simulink model "Solver"  (R2016b)
settings: Solver=ode4  StartTime=0.0  StopTime=Inf  FixedStep=base_dT  RelTol=1e-3
values from neighbouring files (symbols this model uses):
  base_dT = Simulink.Parameter    [SolverInit.m]
  E2C_bEgoFol = Simulink.Parameter    [SolverInit.m]
  E2C_bUseCollo = Simulink.Parameter    [SolverInit.m]
  E2C_c2_dTB = Simulink.Parameter    [SolverInit.m]
  E2C_c_dTB = Simulink.Parameter    [SolverInit.m]
  E2C_d_HDW1 = Simulink.Parameter    [SolverInit.m]
  E2C_d_HDW2 = Simulink.Parameter    [SolverInit.m]
  E2C_DeltaT = Simulink.Parameter    [SolverInit.m]
  E2C_df_term = Simulink.Parameter    [SolverInit.m]
  E2C_dz_term = Simulink.Parameter    [SolverInit.m]
  E2C_Max_iter = Simulink.Parameter    [SolverInit.m]
  E2C_t_HDW1 = Simulink.Parameter    [SolverInit.m]
  E2C_t_HDW2 = Simulink.Parameter    [SolverInit.m]
  E2C_T_TB_thr = Simulink.Parameter    [SolverInit.m]
  E2C_tiSolverPeriod_C = Simulink.Parameter    [SolverInit.m]
  E2C_U_max = Simulink.Parameter    [SolverInit.m]
  E2C_U_min = Simulink.Parameter    [SolverInit.m]
  E2C_V_max = Simulink.Parameter    [SolverInit.m]
  E2C_V_min = Simulink.Parameter    [SolverInit.m]
  E2C_w_delta_u = Simulink.Parameter    [SolverInit.m]
  E2C_w_epsilon_lin = Simulink.Parameter    [SolverInit.m]
  E2C_weight_TTB = Simulink.Parameter    [SolverInit.m]
  Inp_mf_exh_par = Simulink.Parameter    [SolverInit.m]
  Inp_t_eu_par = Simulink.Parameter    [SolverInit.m]
  NP_trial = Simulink.Parameter    [SolverInit.m]
  t_EndSimulation = Simulink.Parameter    [SolverInit.m]
  t_StartSimulation = Simulink.Parameter    [SolverInit.m]
libraries: simulink x3, dspsigops x2
(part 2 of 2)

== matlab function Solver/QP Runner/MATLAB Function - MPC ==
  data: NP input; v_ input; p_ input; T_TB_ input; U_OUTPUT output; v_lead_s input; p_lead input; v_lead input; V_OUTPUT output double; z_laststep input size=[41 1]; z_new output size=[41 1]; w_epsilon input; weight_TTB input; iA0 input boolean size=[NP_trial*6+2,1] [1..250]; t_StartSimulation input; V_lim input; U_lim input; d_HDW input; t_HDW input; w_epsilon_lin input; T_TB_thr input; EgoFol input; UseCollo input; c_dTB input; c2_dTB input; w_delta_u input; t_ input; iA1 output; Inp_mf_exh_par parameter; Inp_t_eu_par parameter; v_0 output size=[40 1]; TTB_0 output size=[40 1]; f_nonl_new output; delta_f output size=[1 1]
function [U_OUTPUT,V_OUTPUT,z_new,iA1,v_0,TTB_0,f_nonl_new,delta_f]    = ...
    NLMPC_TB_Intern_Fcn(NP,v_,p_,T_TB_,v_lead_s,p_lead,v_lead,z_laststep,...
    w_epsilon,weight_TTB,iA0,t_StartSimulation,V_lim,U_lim,d_HDW,t_HDW,w_epsilon_lin,T_TB_thr,EgoFol,UseCollo,...
    c_dTB,c2_dTB,w_delta_u,t_,...
    Inp_mf_exh_par,Inp_t_eu_par)
% 06/29
% change tau_{TB} to c_dTB/(meu+c2_dTB)

%%
% ------------ Load maps  ---------------------------------
Inp.Vspeed = [0:0.1:30]; 
% delta_v = 0.4 does not work!
Inp.Acce = [-6:0.1:6]'; % repmat([-6:0.1:6]',1,351);
Inp.mf_exh = Inp_mf_exh_par; % (1:4:end,1:2:end);
Inp.t_eu = Inp_t_eu_par; % (1:4:end,1:2:end);
% coder.extrinsic('quadprog'); 
% % Option 2:
% % do not use collocation!
% 
if true

%t_ = 0.0;  % not used in testing case. 

assert (NP <= 50);
% assert (NP_trial <= 50);

% persistent PARS
PARS.NP = 40;
PARS.dT = 1;
PARS.weight_a = 1;
PARS.ConstraintCase = 'soft'; % or 'hard' is the same
PARS.t_StartSimulation = t_StartSimulation;

% % ------------ parameters ----------------------------------------------
PARS.V_lim = V_lim;   % inputs from matlab
PARS.U_lim = U_lim;   % inputs from matlab
PARS.d_HDW = d_HDW;   % inputs from matlab
PARS.t_HDW = t_HDW;   % inputs from matlab
PARS.w_epsilon_lin = w_epsilon_lin;
PARS.w_epsilon = w_epsilon;
PARS.T_TB_thr = T_TB_thr;   % 240
PARS.c_dTB = c_dTB;   %3.3
PARS.c2_dTB = c2_dTB;
PARS.w_delta_u = w_delta_u;   % cost on delta_u, originally 0



n = 3; % length(x_)
m = 1; % size(u_past);
Ndec = n + m*(PARS.NP) +1; % [x_,u_opt,t_]
Nz = 3*PARS.NP+1; % z=[du(0),...du(NP-1),dv(1),...,dv(NP),dT(1),...,dT(NP),d_epsilon]



% % ------------ Preview ------------------------------------------------


v_ref = [v_lead_s(1:PARS.NP);v_lead_s(PARS.NP)];
if abs(v_lead-v_ref(1))>1e-6
v_ref(1) = v_lead;
end

z_new = zeros(41,1);

    
acce_ref = (v_ref(2:end)-v_ref(1:end-1))/PARS.dT;
dist_ref = zeros(PARS.NP+1,1);
% coder.varsize('dist_ref', [50,1]); % this is the preview

% initialize

x_ = [v_,p_,T_TB_]';
%coder.extrinsic('linprog'); 
% coder.extrinsic('qinterp2');
% coder.extrinsic('qinterp2_eval');
% coder.extrinsic('tic')
% coder.extrinsic('toc')

% ------------ If do not start optimization -------------------------
if EgoFol==0 || t_<=t_StartSimulation
    U_OUTPUT = 0;
    U_OUTPUT = min(PARS.U_lim(2),(v_lead-v_)/PARS.dT); % track the lead speed% acce_ref(1);
    V_OUTPUT = 0;
    V_OUTPUT = v_ref(1);
    iA1 = false(242,1);     % false(40*4+40*2+2,1);
    z_new = [ones(40,1);0];
    v_0 = v_ref(1:40);
    TTB_0 = 150+0*v_0;
    f_nonl_new = 100;
    delta_f = 0;
else
    % ------------ CREATE DISTANCE BOUNDS ---------------------------------

    dist_ref(1) = p_lead;
    A3t = zeros(PARS.NP);
    for i=1:PARS.NP
        A3t(i:PARS.NP,i) = [1:PARS.NP-i+1]-0.5;
    end
    Aineq3 = [ [PARS.dT:PARS.dT:PARS.NP*PARS.dT]', ones(PARS.NP,1), zeros(PARS.NP,n-2), A3t*PARS.dT^2 ,zeros(PARS.NP,1)];
    dist_ref(2:PARS.NP+1) = Aineq3*[[v_ref(1);p_lead;0];acce_ref;0];
    dist_hi_ref = dist_ref - PARS.d_HDW(1);
    dist_lo_ref = dist_ref - PARS.d_HDW(2);

    % --------------- Optimization reference ------------------------------
    z_cur_2 = z_laststep;    % z_cur_2 should be the guessed z_curr step, from either z_curr-1 or from last sqp iteration.
    
    z_cur = zeros(45,1);      % zeros(3+40+1+1,1);
    z_cur = [x_;z_cur_2(1:PARS.NP);t_;z_cur_2(PARS.NP+1)];
    
    % ----------- reference Acceleration -----------------------------------------
    % if max(TTB_laststep)<=150.1 && min(TTB_laststep)>=149.9
    u_opt = zeros(40,1);
    u_opt = z_cur_2(1:PARS.NP);
    u_opt(u_opt>PARS.U_lim(2)) = PARS.U_lim(2);
    u_opt(u_opt<PARS.U_lim(1)) = PARS.U_lim(1);
    z_cur_2(1:PARS.NP) = u_opt;
    v_opt = zeros(40,1);
    % v_opt = v(curr+1:curr+NP)
    Aineq1 = [ones(PARS.NP,1),zeros(PARS.NP,n-1),PARS.dT*tril(ones(PARS.NP,PARS.NP),0),zeros(PARS.NP,1)];
    v_opt = Aineq1*z_cur(1:n+PARS.NP+1);
    v_opt(v_opt<PARS.V_lim(1))=PARS.V_lim(1);
    v_opt(v_opt>PARS.V_lim(2))=PARS.V_lim(2);

    u_opt = (v_opt-[v_;v_opt(1:40-1)])/PARS.dT;
    u_opt(u_opt>PARS.U_lim(2)) = PARS.U_lim(2);
    u_opt(u_opt<PARS.U_lim(1)) = PARS.U_lim(1);
    v_0 = zeros(40,1); 
    v_0(1:PARS.NP) = [max(min(v_,PARS.V_lim(2)),PARS.V_lim(1));v_opt(1:PARS.NP-1)];  % nominal v at t(curr:curr+NP-1)
    
    % ------------ Hession ------------ 
    % add cost on sum(delta_u) 06/17/2019
    H_delta_u = zeros(PARS.NP+1);
    H_delta_u(1,1) = 1 *2*PARS.w_delta_u;
    H_delta_u(PARS.NP,PARS.NP) = 1 *2*PARS.w_delta_u;
    for i = 2:PARS.NP-1
        H_delta_u(i,i) = 2 * 2*PARS.w_delta_u;
        H_delta_u(i-1,i) = -1 * 2*PARS.w_delta_u;
        H_delta_u(i,i-1) = -1 * 2*PARS.w_delta_u;
    end
    H_delta_u(PARS.NP-1,PARS.NP) = -1 * 2*PARS.w_delta_u;
    H_delta_u(PARS.NP,PARS.NP-1) = -1 * 2*PARS.w_delta_u;
    
    % ------------ calculate the cost before opt ------------ 
    ind1 = 0.0*zeros(40,1); %(0*v_0)*zeros(1,4);
    ind2 = 0.0*zeros(40,1);
    ind3 = 0.0*zeros(40,1);
    ind4 = 0.0*zeros(40,1);
    dfxi = 0.0*zeros(40,1); % (0*v_0)*zeros(1,2);
    dfyi = 0.0*zeros(40,1); % (0*v_0)*zeros(1,2);
    flagIn = zeros(40,1); % 0*v_0;
    % [ind,dfxy,flagIn] = qinterp2(Inp.Vspeed, Inp.Acce, v_0, u_opt, 2);
    %% This section is qinterp2.m
%     X = Inp.Vspeed;
%     Y = Inp.Acce;
    xi = v_0;
    yi = u_opt;
    librarySize = [0 0];
    librarySize = [length(Inp.Acce),length(Inp.Vspeed)];
    ndx = 0.0;  ndy = 0.0;
    ndx = 1/(Inp.Vspeed(1,2)-Inp.Vspeed(1,1));    
    ndy = 1/(Inp.Acce(2,1)-Inp.Acce(1,1));
    % Begin mapping xi and yi vectors onto index space by subtracting library
    % array minima and scaling to index spacing
    xi(xi>=Inp.Vspeed(1,end)) = Inp.Vspeed(1,end)-1e-8*(Inp.Vspeed(1,end)-Inp.Vspeed(1,1));
    yi(yi>=Inp.Acce(end,1)) = Inp.Acce(end,1)-1e-8*(Inp.Acce(end,1)-Inp.Acce(1,1));

    xi = (xi - Inp.Vspeed(1,1))*ndx;       yi = (yi - Inp.Acce(1,1))*ndy;
    fxi = floor(xi)+1;  fyi = floor(yi)+1;   % x_i and y_i
    dfxi = xi-fxi+1;    dfyi = yi-fyi+1;     % Location in unit square

    % flagIn determines whether the requested location is inside of the
    % library arrays
    flagIn = fxi>0 & fxi<librarySize(2) & ~isnan(fxi) &...
        fyi>0 & fyi<librarySize(1) & ~isnan(fyi);
%     if min(flagIn)==0
%         1+1
%         flagIn
%     end
    % Toss all out-of-bounds variables now to save time
    fxi = fxi(flagIn); fyi = fyi(flagIn);
    dfxi = dfxi(flagIn); dfyi = dfyi(flagIn);

    % Find bounding vertices
    ind1 = fyi + librarySize(1)*(fxi-1);     % Indices of (  x_i  ,  y_i  )
    ind2 = fyi + librarySize(1)*fxi;         % Indices of ( x_i+1 ,  y_i  )
    ind3 = fyi + 1 + librarySize(1)*fxi;     % Indices of ( x_i+1 , y_i+1 )
    ind4 = fyi + 1 + librarySize(1)*(fxi-1); % Indices of (  x_i  , y_i+1 )


    flagIn = double(flagIn);

    %%

    TTB_0 = zeros(40,1);
    TTB_0(1:PARS.NP) = [x_(3); zeros(PARS.NP-1,1)];
    meu_0 = zeros(40,1);
    Tin_0 = zeros(40,1);

    % meu_0 = qinterp2_eval(Inp.mf_exh, ind,dfxy,flagIn);
    % Tin_0 = qinterp2_eval(Inp.t_eu, ind,dfxy,flagIn);
    %% This is for qinterp2_eval.m
    Z = Inp.mf_exh; 
    Zi = 0.0*ind1;
    Zi(find(flagIn==1)) = Z(ind1).*(1-dfxi).*(1-dfyi) + ...
        Z(ind2).*dfxi.*(1-dfyi) + ...
        Z(ind4).*(1-dfxi).*dfyi + ...
        Z(ind3).*dfxi.*dfyi;
    meu_0 = Zi;
    % derivatives
%     p_meu_p_u = qinterp2_eval(Inp.mf_exh_pu, ind,dfxy,flagIn);
%     p_meu_p_x = qinterp2_eval(Inp.mf_exh_px, ind,dfxy,flagIn);
    p_meu_p_u = 0.0*v_0;
    p_meu_p_x = 0.0*v_0;
    p_meu_p_u = (Z(ind4)-Z(ind1)).*(1-dfxi)*ndy + ...
        (Z(ind3)-Z(ind2)).*(dfxi)*ndy;
    p_meu_p_x = (Z(ind2)-Z(ind1))*ndx.*(1-dfyi) + ...
        (Z(ind3)-Z(ind4))*ndx.*(dfyi);

    Z = Inp.t_eu; 
    Zi(find(flagIn==1)) = Z(ind1).*(1-dfxi).*(1-dfyi) + ...
        Z(ind2).*dfxi.*(1-dfyi) + ...
        Z(ind4).*(1-dfxi).*dfyi + ...
        Z(ind3).*dfxi.*dfyi;
    Tin_0 = Zi;
    % derivatives
%     p_Teu_p_u = qinterp2_eval(Inp.t_eu_pu, ind,dfxy,flagIn);
%     p_Teu_p_x = qinterp2_eval(Inp.t_eu_px, ind,dfxy,flagIn);
    p_Teu_p_u = 0.0*v_0;
    p_Teu_p_x = 0.0*v_0;
    p_Teu_p_u = (Z(ind4)-Z(ind1)).*(1-dfxi)*ndy + ...
        (Z(ind3)-Z(ind2)).*(dfxi)*ndy;
    p_Teu_p_x = (Z(ind2)-Z(ind1))*ndx.*(1-dfyi) + ...
        (Z(ind3)-Z(ind4))*ndx.*(dfyi);

    %%
%     for i = 1:PARS.NP-1
%         TTB_0(i+1,1) = TTB_0(i,1) + PARS.dT.*meu_0(i,1)/PARS.c_dTB.*(Tin_0(i,1)-TTB_0(i,1));
%     end
    for i = 1:PARS.NP-1
        TTB_0(i+1,1) = TTB_0(i,1) + PARS.dT.*(meu_0(i,1)+PARS.c2_dTB)/PARS.c_dTB.*(Tin_0(i,1)-TTB_0(i,1));
    end
    
    f_nonl = 0; % compute the actual cost value
    f_nonl = u_opt'*eye(PARS.NP)*u_opt + ...
        (1e-3*weight_TTB)*sum(double(TTB_0<PARS.T_TB_thr).*(TTB_0-PARS.T_TB_thr).^2) + ...
        PARS.w_epsilon*(z_cur_2(PARS.NP+1))^2 + ...
        PARS.w_epsilon_lin*(z_cur_2(PARS.NP+1)) + ...
        0.5*u_opt'*H_delta_u(1:PARS.NP,1:PARS.NP)*u_opt;
    
    % ------------ Create NLMPC Aeq,Beq ------------------------------------
    Aeq = zeros(n, Ndec);
    beq = zeros(n, 1);
    Aeq(1:n, 1:n) = eye(n);
    beq(1:n) = x_;

    % ------------ Create NLMPC Aineq,Bineq ------------------------------------
    Aineq1 = [ones(PARS.NP,1),zeros(PARS.NP,n-1),PARS.dT*tril(ones(PARS.NP,PARS.NP),0),zeros(PARS.NP,1)];
    bineq1 = V_lim(2)-0.001+zeros(PARS.NP,1);
    Aineq2 = -Aineq1;
    bineq2 = -(V_lim(1)-0.001)+zeros(PARS.NP,1);
    % Aineq3 already defined above
    bineq3 = dist_hi_ref(2:PARS.NP+1);
    Aineq4 = -Aineq3;
    bineq4 = -( dist_lo_ref(2:PARS.NP+1) );
    Aineq5 = [];
    bineq5 = [];

    
%     AINEQ = [[Aineq1;Aineq2;Aineq3+PARS.t_HDW(1)*Aineq1;Aineq4-PARS.t_HDW(2)*Aineq1;Aineq5],...
%         [-1e-5*ones(2*length(Aineq1(:,1)),1);-ones(2*length(Aineq1(:,1)),1);zeros(length(bineq5),1)]];
%     BINEQ = [bineq1;bineq2;bineq3;bineq4;bineq5];

    % ----------- Create NLMPC lb,ub -----------------------------------------
    lb = zeros(3 + 40 +1,1);
    ub = zeros(3 + 40 +1,1);
    lb(end) = t_;
    ub(end) = t_;
    lb(1:3) = x_;
    ub(1:3) = x_;
    lb(1+3:3+40) = PARS.U_lim(1);
    ub(1+3:3+40) = PARS.U_lim(2);

    % ----------- Create Initial guess -----------------------------------------
%     if iter ==0
%         z_last = zeros(40+1,1);  %initial guess.  n+PARS.NP+1
%         for i = 1:40
%             z_last(i) = interp1([-0.1;t_laststep;20000],[0;u_laststep;0],t_+i-1);
%         end
%         z_last(40+1) = 0;  
%         z_laststep = z_last; 
%     else
%         % z_laststep = z_laststep; % in the same sqp, not same qp.
%     end
    % --------------- Optimization reference ------------------------------
    Hession_f1 = 2* 1*diag([ones(1,PARS.NP), PARS.w_epsilon ]) + H_delta_u; % a^2+epsilon^2part
    
    

    % ----------- calculate gradient ------------------
    % grad_z(f)
    % we need 

    

%     % ---------------------finite differentence calculating gradiant ---------------
%     du = 0.001;
%     delta_u = du*ones(40,1);  % perturbation of u
%     V_pert = zeros(40,40);
%     % V_pert = v_{0:NP-1}(u^0+du(0)),v_{0:NP-1}(u^0+du(1)),...,v_{0:NP-1}(u^0+du(NP-1))
%     % first column, perturb du(0),affect 2:NP;
%     % second column, perturb du(1),affect 3:NP;
%     % last column, perturb du(1)
%     V_pert = [[1,zeros(1,n+PARS.NP-1)];Aineq1(1:PARS.NP-1,1:n+PARS.NP)]*[x_*(1+0*u_opt');u_opt*(1+0*u_opt')+diag(delta_u)];
%     V_pert=max(V_pert,0);
%     V_pert=min(V_pert,30);
%     V_ppert = V_pert*2- v_0*(1+0*v_0');
%     V_ppert = v_{0:NP-1}(u^0+2du(0)),v_{0:NP-1}(u^0+2du(1)),...,v_{0:NP-1}(u^0+2du(NP-1))
%         TTB_pert = zeros(40,40);
%         TTB_pert = TTB_0*(1+0*TTB_0');  % upper right small triangle is equal to TTB_0.
% 
%         for i = 1:PARS.NP-1
%             u_pert = u_opt*0;
%             u_pert = u_opt;
%             u_pert(i) = u_pert(i)+du;
%             ind_i = zeros(40-i+1,4); %(0*v_0)*zeros(1,4);
%             dfxy_i = zeros(40-i+1,2); % (0*v_0)*zeros(1,2);
%             flagIn_i = zeros(40-i+1,1); % 0*v_0;
% 
%             [ind_i,dfxy_i,flagIn_i] = qinterp2(Inp.Vspeed, Inp.Acce, V_pert(i:PARS.NP,i), u_pert(i:PARS.NP), 2);
%             meu_i = zeros(40-i+1,1);
%             meu_i = qinterp2_eval(Inp.mf_exh, ind_i,dfxy_i,flagIn_i );
%             Tin_i = zeros(40-i+1,1);
%             Tin_i = qinterp2_eval(Inp.t_eu, ind_i,dfxy_i,flagIn_i );
%             for j = i:PARS.NP-1
%                 TTB_pert(j+1,i) = TTB_pert(j,i)+PARS.dT.*meu_i(j-(i-1))/3.3.*(Tin_i(j-(i-1))-TTB_pert(j,i));
%             end
%         end
%         grad_f2_p1 = [0*delta_u;0]*(0*delta_u)';
%         grad_f2_p1(1:PARS.NP,1:PARS.NP) = ((TTB_pert-TTB_0*(1+0*TTB_0'))/du)';
%         grad_f2_p2 = 0*delta_u;
%         grad_f2_p2 = (1e-3*weight_TTB)*(TTB_0-240).*(TTB_0<240);
%         grad_f2 = [0*delta_u;0];
%         grad_f2 = grad_f2_p1*grad_f2_p2;
%         Hession_f2 = [0*delta_u;0]*[0*delta_u;0]';
%         Hession = Hession_f1+Hession_f2;
%         grad_f1 = Hession_f1*z_cur_2;
%         grad_f = 0*grad_f1;
%         grad_f = grad_f1 + grad_f2;
%     
    % --------------------- direct calculating gradiant ---------------
    
    Hession_f2 = [0*v_0;0]*[0*v_0;0]';
    Hession = Hession_f1 + Hession_f2; %0.5*z'*H*z!!
    grad_f1 = Hession_f1*z_cur_2 + [0*v_0;PARS.w_epsilon_lin];
    


    %%
%     d_TTB_plus_d_z = PARS.dT/PARS.c_dTB*( p_Teu_p_u.*meu_0 + (Tin_0-TTB_0).*p_meu_p_u ); % PARS.c_dTB = 3.3
%     d_TTB_plus_d_z(PARS.NP) = 0;
%     p_TTB_plus_p_x = PARS.dT/PARS.c_dTB*( p_Teu_p_x.*meu_0 + (Tin_0-TTB_0).*p_meu_p_x );
%     p_TTB_plus_p_x(PARS.NP) = 0;
%     p_TTB_plus_p_TTB = 1-PARS.dT/PARS.c_dTB*meu_0;
%     p_TTB_plus_p_TTB(PARS.NP) = 0;
    
    d_TTB_plus_d_z = PARS.dT*( p_Teu_p_u.*(meu_0+PARS.c2_dTB)/PARS.c_dTB + (Tin_0-TTB_0).*p_meu_p_u/PARS.c_dTB ); % PARS.c_dTB = 3.3
    d_TTB_plus_d_z(PARS.NP) = 0;
    p_TTB_plus_p_x = PARS.dT*( p_Teu_p_x.*(meu_0+PARS.c2_dTB)/PARS.c_dTB + (Tin_0-TTB_0).*p_meu_p_x/PARS.c_dTB );
    p_TTB_plus_p_x(PARS.NP) = 0;
    p_TTB_plus_p_TTB = 1-PARS.dT/PARS.c_dTB*(meu_0+PARS.c2_dTB);
    p_TTB_plus_p_TTB(PARS.NP) = 0;
    
    
    d_TTB_d_z = 0*v_0*[0*v_0;0]'; % NP*(NP+1)
    for i = 1:PARS.NP-1 % i is the row
        d_TTB_d_z(i+1,i) = d_TTB_plus_d_z(i);
    end
    
    for i = 3:PARS.NP % i is the row
        d_TTB_d_z(i,1:i-2) = PARS.dT*p_TTB_plus_p_x(i-1) + d_TTB_d_z(i-1,1:i-2)*p_TTB_plus_p_TTB(i-1);
    end
    
    grad_f2_p2 = 2*(1e-3*weight_TTB)*(TTB_0-240).*(double(TTB_0<240));  % changed to ("2*") 06062019
    grad_f2 = (grad_f2_p2'*d_TTB_d_z)';
    
    grad_f = 0*grad_f1;
    grad_f = grad_f1 + grad_f2;
    
    % ------------- optimize --------------------------------
    
    c_f = grad_f;
    [L,~] = chol(Hession+1e-10*eye(PARS.NP+1),'lower');
    Linv = (L)\eye(PARS.NP+1);
    opt = mpcqpsolverOptions;
    
    A_qp = zeros(242,41);
    b_qp = zeros(242,1);
%     A_qp = zeros(length(BINEQ)+2*NP_par+2, NP_par+1);
%     b_qp = zeros(length(BINEQ)+2*NP_par+2, 1);
    
%     A_qp = [[AINEQ(1:40*4,3+1:3+40),AINEQ(1:40*4,3+40+2)]; eye(40+1); -eye(40+1)];
%     % b_qp = [BINEQ(1:4*40) - AINEQ(:,1:n)*x_; [ub(n+1:n+40);1000]; [-lb(n+1:n+40);-0]];
%     b_qp = [BINEQ(1:4*40) - AINEQ(:,1:n)*x_; [ub(3+1:3+40);1000]; [-lb(3+1:3+40);-0]];
%     % A_qp*(z_cur+d_z)<=b_qp <-> A_qp*(d_z) <=b_qp - A_qp*z_cur
    A_qp = [[[Aineq1(:, 3+1:3+40);Aineq2(:, 3+1:3+40);Aineq3(:,3+1:3+40)+PARS.t_HDW(1)*Aineq1(:,3+1:3+40);Aineq4(:,3+1:3+40)-PARS.t_HDW(2)*Aineq1(:,3+1:3+40)],...
        [-1e-5*ones(2*length(Aineq1(:,1)),1);-ones(2*length(Aineq1(:,1)),1);zeros(0,1)]]; eye(40+1); -eye(40+1)];
    b_qp = [[bineq1;bineq2;bineq3;bineq4] - [Aineq1(:, 1:n);Aineq2(:, 1:n);Aineq3(:, 1:n)+PARS.t_HDW(1)*Aineq1(:,1:n);Aineq4(:, 1:n)-PARS.t_HDW(2)*Aineq1(:,1:n)]*x_; ...
        [PARS.U_lim(2)+zeros(40,1);9000]; [-PARS.U_lim(1)+zeros(40,1);-0]];
    % max(max(abs(b_qp -[BINEQ(1:4*40) - AINEQ(:,1:n)*x_; [ub(3+1:3+40);1000]; [-lb(3+1:3+40);-0]])))
    
    Aeq_qp = [];
    beq_qp = zeros(0,1);
    % iA0 = false(size(b_qp));
    
    iA1 = false(40*4+40*2+2,1);
    status = 0; % [z_cur_2,status,iA1,~]
    d_z = 0*z_cur_2;  % NP+1
    %[d_z,~,~,~] = quadprog(Hession+1e-10*eye(PARS.NP+1), c_f, A_qp, b_qp-A_qp*z_cur_2 ,Aeq_qp,beq_qp,[],[],u_opt);
    %iA1 = false(40*4+40*2+2,1);
    % 2015b mpcqpsolver
    [d_z,status,iA1,~] = mpcqpsolver(Linv,c_f,-(A_qp),-(b_qp-A_qp*z_cur_2),Aeq_qp,beq_qp,iA0,opt); 
    %A_mpc*x>=b_mpc!
    %works!
    z_cur_2_new = zeros(41,1);

    if length(iA1) ~= 40*4+40*2+2
        iA1 = false(40*4+40*2+2,1);
    end
    if length(d_z) ~= 41
        d_z = zeros(41,1);
    end
    
    % -------------- line search backtracking -----------------------------
    % f_nonl
    alpha = 0.0;
    alpha = 2.0;
    alpha_min = 0.0;
    alpha_min = 2^(-10);
    f_nonl_new = f_nonl + 100;
    
    if max(-(b_qp-A_qp*z_cur_2))<1e-6 % && max(abs(beq_qp))<1e-6  % then zeros(NP+1,1) is a feasible solution
        % perform line search
        while f_nonl_new>f_nonl && alpha > alpha_min
            if alpha < 1.5
                f_nonl = min(f_nonl_new,f_nonl); % lowest cost ever since
            end
            alpha = 0.5*alpha;
            z_cur_2_new = z_cur_2 + alpha*d_z;
            z_cur = zeros(45,1);     % zeros(3+40+1+1,1);
            u_opt = zeros(40,1);
            u_opt = z_cur_2_new(1:PARS.NP);
            u_opt(u_opt>PARS.U_lim(2)) = PARS.U_lim(2);
            u_opt(u_opt<PARS.U_lim(1)) = PARS.U_lim(1);
            z_cur_2_new(1:PARS.NP) = u_opt;
            z_cur = [x_;z_cur_2_new(1:PARS.NP);t_;z_cur_2_new(PARS.NP+1)];

            v_opt = zeros(40,1);
            % v_opt = v(curr+1:curr+NP)
            v_opt = Aineq1*z_cur(1:n+PARS.NP+1);
            v_opt(v_opt<PARS.V_lim(1))=PARS.V_lim(1);
            v_opt(v_opt>PARS.V_lim(2))=PARS.V_lim(2);
            u_opt = (v_opt-[v_;v_opt(1:40-1)])/PARS.dT;
            u_opt(u_opt>PARS.U_lim(2)) = PARS.U_lim(2);
            u_opt(u_opt<PARS.U_lim(1)) = PARS.U_lim(1);
            z_cur_2_new(1:PARS.NP) = u_opt;

            v_0 = zeros(40,1); 
            v_0(1:PARS.NP) = [max(min(v_,PARS.V_lim(2)),PARS.V_lim(1));v_opt(1:PARS.NP-1)];

            % f_nonl is the cost before this step.
            % -------------- compute new costs ----------------------------
            ind1 = 0.0*zeros(40,1); %(0*v_0)*zeros(1,4);
            ind2 = 0.0*zeros(40,1);
            ind3 = 0.0*zeros(40,1);
            ind4 = 0.0*zeros(40,1);
            dfxi = 0.0*zeros(40,1); % (0*v_0)*zeros(1,2);
            dfyi = 0.0*zeros(40,1); % (0*v_0)*zeros(1,2);
            flagIn = zeros(40,1); % 0*v_0;
            % [ind,dfxy,flagIn] = qinterp2(Inp.Vspeed, Inp.Acce, v_0, u_opt, 2);
            %% This section is qinterp2.m
%             X = Inp.Vspeed;
%             Y = Inp.Acce;
            xi = v_0;
            yi = u_opt;
            librarySize = [0 0];
            librarySize = [length(Inp.Acce),length(Inp.Vspeed)];
            ndx = 0.0;  ndy = 0.0;
            ndx = 1/(Inp.Vspeed(1,2)-Inp.Vspeed(1,1));    
            ndy = 1/(Inp.Acce(2,1)-Inp.Acce(1,1));
            % Begin mapping xi and yi vectors onto index space by subtracting library
            % array minima and scaling to index spacing
            xi(xi>=Inp.Vspeed(1,end)) = Inp.Vspeed(1,end)-1e-8*(Inp.Vspeed(1,end)-Inp.Vspeed(1,1));
            yi(yi>=Inp.Acce(end,1)) = Inp.Acce(end,1)-1e-8*(Inp.Acce(end,1)-Inp.Acce(1,1));

            xi = (xi - Inp.Vspeed(1,1))*ndx;       yi = (yi - Inp.Acce(1,1))*ndy;
            fxi = floor(xi)+1;  fyi = floor(yi)+1;   % x_i and y_i
            dfxi = xi-fxi+1;    dfyi = yi-fyi+1;     % Location in unit square
            
            % flagIn determines whether the requested location is inside of the
            % library arrays
            flagIn = double(fxi>0 & fxi<librarySize(2) & ~isnan(fxi) & fyi>0 & fyi<librarySize(1) & ~isnan(fyi));
            % Toss all out-of-bounds variables now to save time
            fxi = fxi(flagIn==1); fyi = fyi(flagIn==1);
            dfxi = dfxi(flagIn==1); dfyi = dfyi(flagIn==1);
            % Find bounding vertices
            ind1 = fyi + librarySize(1)*(fxi-1);     % Indices of (  x_i  ,  y_i  )
            ind2 = fyi + librarySize(1)*fxi;         % Indices of ( x_i+1 ,  y_i  )
            ind3 = fyi + 1 + librarySize(1)*fxi;     % Indices of ( x_i+1 , y_i+1 )
            ind4 = fyi + 1 + librarySize(1)*(fxi-1); % Indices of (  x_i  , y_i+1 )
            % outputs
%             ind = [ind1,ind2,ind3,ind4];
%             dfxy = [dfxi,dfyi];
            flagIn = double(flagIn);

            %%
            TTB_0 = zeros(40,1);
            TTB_0(1:PARS.NP) = [x_(3); zeros(PARS.NP-1,1)];
            meu_0 = zeros(40,1);
            Tin_0 = zeros(40,1);
            % meu_0 = qinterp2_eval(Inp.mf_exh, ind,dfxy,flagIn);
            % Tin_0 = qinterp2_eval(Inp.t_eu, ind,dfxy,flagIn);
            %% This is for qinterp2_eval.m
            Z = Inp.mf_exh; 
            Zi = 0.0*ind1;
            Zi(find(flagIn==1)) = Z(ind1).*(1-dfxi).*(1-dfyi) + ...
                Z(ind2).*dfxi.*(1-dfyi) + ...
                Z(ind4).*(1-dfxi).*dfyi + ...
                Z(ind3).*dfxi.*dfyi;
            meu_0 = Zi;
            Z = Inp.t_eu; 
            Zi(find(flagIn==1)) = Z(ind1).*(1-dfxi).*(1-dfyi) + ...
                Z(ind2).*dfxi.*(1-dfyi) + ...
                Z(ind4).*(1-dfxi).*dfyi + ...
                Z(ind3).*dfxi.*dfyi;
            Tin_0 = Zi;

            %%
%             for i = 1:PARS.NP-1
%                 TTB_0(i+1,1) = TTB_0(i,1) + PARS.dT.*meu_0(i,1)/PARS.c_dTB.*(Tin_0(i,1)-TTB_0(i,1));
%             end
            for i = 1:PARS.NP-1
                TTB_0(i+1,1) = TTB_0(i,1) + PARS.dT.*(meu_0(i,1)+PARS.c2_dTB)/PARS.c_dTB.*(Tin_0(i,1)-TTB_0(i,1));
            end
            
            f_nonl_new = 0; % compute the actual cost value
            f_nonl_new = u_opt'*eye(PARS.NP)*u_opt + ...
                (1e-3*weight_TTB)*sum(double(TTB_0<PARS.T_TB_thr).*(TTB_0-PARS.T_TB_thr).^2) + ...
                PARS.w_epsilon*(z_cur_2(PARS.NP+1))^2 +...
                PARS.w_epsilon_lin*(z_cur_2(PARS.NP+1))+ ...
                0.5*u_opt'*H_delta_u(1:PARS.NP,1:PARS.NP)*u_opt;
            
            
         
    
            [f_nonl,f_nonl_new];
            % disp('improvement = ');
            [f_nonl-f_nonl_new];
    
        end % while
    else
        z_cur_2_new = z_cur_2 + 1*d_z;
            z_cur = zeros(3+40+1+1,1);
            u_opt = zeros(40,1);
            u_opt = z_cur_2_new(1:PARS.NP);
            u_opt(u_opt>PARS.U_lim(2)) = PARS.U_lim(2);
            u_opt(u_opt<PARS.U_lim(1)) = PARS.U_lim(1);
            z_cur_2_new(1:PARS.NP) = u_opt;
            z_cur = [x_;z_cur_2_new(1:PARS.NP);t_;z_cur_2_new(PARS.NP+1)];

            v_opt = zeros(40,1);
            % v_opt = v(curr+1:curr+NP)
            v_opt = Aineq1*z_cur(1:n+PARS.NP+1);
            v_opt(v_opt<PARS.V_lim(1))=PARS.V_lim(1);
            v_opt(v_opt>PARS.V_lim(2))=PARS.V_lim(2);
            u_opt = (v_opt-[v_;v_opt(1:40-1)])/PARS.dT;
            u_opt(u_opt>PARS.U_lim(2)) = PARS.U_lim(2);
            u_opt(u_opt<PARS.U_lim(1)) = PARS.U_lim(1);
            z_cur_2_new(1:PARS.NP) = u_opt;

            v_0 = zeros(40,1); 
            v_0(1:PARS.NP) = [max(min(v_,PARS.V_lim(2)),PARS.V_lim(1));v_opt(1:PARS.NP-1)];

            % f_nonl is the cost before this step.
            % -------------- compute new costs ----------------------------
            ind1 = 0.0*zeros(40,1); %(0*v_0)*zeros(1,4);
            ind2 = 0.0*zeros(40,1);
            ind3 = 0.0*zeros(40,1);
            ind4 = 0.0*zeros(40,1);
            dfxi = 0.0*zeros(40,1); % (0*v_0)*zeros(1,2);
            dfyi = 0.0*zeros(40,1); % (0*v_0)*zeros(1,2);
            flagIn = zeros(40,1); % 0*v_0;
            % [ind,dfxy,flagIn] = qinterp2(Inp.Vspeed, Inp.Acce, v_0, u_opt, 2);
            %% This section is qinterp2.m
%             X = Inp.Vspeed;
%             Y = Inp.Acce;
            xi = v_0;
            yi = u_opt;
            librarySize = [0 0];
            librarySize = [length(Inp.Acce),length(Inp.Vspeed)];
            ndx = 0;  ndy = 0;
            ndx = 1/(Inp.Vspeed(1,2)-Inp.Vspeed(1,1));    
            ndy = 1/(Inp.Acce(2,1)-Inp.Acce(1,1));
            % Begin mapping xi and yi vectors onto index space by subtracting library
            % array minima and scaling to index spacing
            xi(xi>=Inp.Vspeed(1,end)) = Inp.Vspeed(1,end)-1e-8*(Inp.Vspeed(1,end)-Inp.Vspeed(1,1));
            yi(yi>=Inp.Acce(end,1)) = Inp.Acce(end,1)-1e-8*(Inp.Acce(end,1)-Inp.Acce(1,1));
            xi = (xi - Inp.Vspeed(1,1))*ndx;       yi = (yi - Inp.Acce(1,1))*ndy;
            fxi = floor(xi)+1;  fyi = floor(yi)+1;   % x_i and y_i
            dfxi = xi-fxi+1;    dfyi = yi-fyi+1;     % Location in unit square
            
            % flagIn determines whether the requested location is inside of the
            % library arrays
            flagIn = double(fxi>0 & fxi<librarySize(2) & ~isnan(fxi) & fyi>0 & fyi<librarySize(1) & ~isnan(fyi));
            % Toss all out-of-bounds variables now to save time
            fxi = fxi(flagIn==1); fyi = fyi(flagIn==1);
            dfxi = dfxi(flagIn==1); dfyi = dfyi(flagIn==1);
            % Find bounding vertices
            ind1 = fyi + librarySize(1)*(fxi-1);     % Indices of (  x_i  ,  y_i  )
            ind2 = fyi + librarySize(1)*fxi;         % Indices of ( x_i+1 ,  y_i  )
            ind3 = fyi + 1 + librarySize(1)*fxi;     % Indices of ( x_i+1 , y_i+1 )
            ind4 = fyi + 1 + librarySize(1)*(fxi-1); % Indices of (  x_i  , y_i+1 )
            % outputs
%             ind = [ind1,ind2,ind3,ind4];
%             dfxy = [dfxi,dfyi];
            flagIn = double(flagIn);

            %%
            TTB_0 = zeros(40,1);
            TTB_0(1:PARS.NP) = [x_(3); zeros(PARS.NP-1,1)];
            meu_0 = zeros(40,1);
            Tin_0 = zeros(40,1);
            % meu_0 = qinterp2_eval(Inp.mf_exh, ind,dfxy,flagIn);
            % Tin_0 = qinterp2_eval(Inp.t_eu, ind,dfxy,flagIn);
            %% This is for qinterp2_eval.m
            Z = Inp.mf_exh; 
            Zi = 0.0*ind1;
            Zi(find(flagIn==1)) = Z(ind1).*(1-dfxi).*(1-dfyi) + ...
                Z(ind2).*dfxi.*(1-dfyi) + ...
                Z(ind4).*(1-dfxi).*dfyi + ...
                Z(ind3).*dfxi.*dfyi;
            meu_0 = Zi;
            Z = Inp.t_eu; 
            Zi(find(flagIn==1)) = Z(ind1).*(1-dfxi).*(1-dfyi) + ...
                Z(ind2).*dfxi.*(1-dfyi) + ...
                Z(ind4).*(1-dfxi).*dfyi + ...
                Z(ind3).*dfxi.*dfyi;
            Tin_0 = Zi;

            %%
%             for i = 1:PARS.NP-1
%                 TTB_0(i+1,1) = TTB_0(i,1) + PARS.dT.*meu_0(i,1)/PARS.c_dTB.*(Tin_0(i,1)-TTB_0(i,1));
%             end
            for i = 1:PARS.NP-1
                TTB_0(i+1,1) = TTB_0(i,1) + PARS.dT.*(meu_0(i,1)+PARS.c2_dTB)/PARS.c_dTB.*(Tin_0(i,1)-TTB_0(i,1));
            end
            
            f_nonl_new = 0; % compute the actual cost value
            f_nonl_new = u_opt'*eye(PARS.NP)*u_opt + ...
                (1e-3*weight_TTB)*sum(double(TTB_0<PARS.T_TB_thr).*(TTB_0-PARS.T_TB_thr).^2) + ...
                PARS.w_epsilon*(z_cur_2(PARS.NP+1))^2 +...
                PARS.w_epsilon_lin*(z_cur_2(PARS.NP+1))+ ...
                0.5*u_opt'*H_delta_u(1:PARS.NP,1:PARS.NP)*u_opt;
            
            
    end %if
    % -------------------------------------------------------------
    
    
    % ------------ CREATE Outputs ---------------------------------
    z_new = z_cur_2_new.*(ones(41,1));
    % output v_0
    % TTB_0
    % f_nonl_new
    delta_f = 0;
    if f_nonl-f_nonl_new>0 % || alpha ==2
        delta_f = f_nonl-f_nonl_new;
    elseif f_nonl-f_nonl_new<=0 && alpha <= alpha_min % means cannot improve even with alpha_min
        z_new = z_cur_2.*(ones(41,1)); % use the last result and will stop
        delta_f = 1;
        % disp('Cannot improve');
    else
        delta_f = 1; % this happens if f_nonl-f_nonl_new<=0 && alpha > alpha_min --> did not do line search
    end
    
    U_OUTPUT = z_new(1); %(v_opt(1)-v_)/PARS.dT; % track the optimal speed
    U_OUTPUT(U_OUTPUT>PARS.U_lim(2)) = PARS.U_lim(2);
    U_OUTPUT(U_OUTPUT<PARS.U_lim(1)) = PARS.U_lim(1);
    if v_+PARS.dT*U_OUTPUT >PARS.V_lim(2)
        U_OUTPUT = (PARS.V_lim(2)-v_)/PARS.dT;
    elseif v_+PARS.dT*U_OUTPUT <PARS.V_lim(1)
        U_OUTPUT = (PARS.V_lim(1)-v_)/PARS.dT;
    end
    
    V_OUTPUT = v_+PARS.dT*U_OUTPUT; % ???? do not know the time step, how to set speed target?
    
    % u_new = u_opt;
    
    
    %%%%%%%%%%%%%%%%%%%%%%%%%%%%%%%%%%%%%%%%%%%%%
% dpttt = toc;
% disp(dpttt);

end

end

== stateflow chart Solver/Solver_Control ==
  state task_sched [parallel]
    settings: executionOrder=1
    state task_hold
    (default) -> (junction 181)
    (junction 181) -> task_hold : {b_doGrad=false;b_doQP=false;b_exitQP=false;b_termQP=false;
        | E2C_stSolve=false;E2C_stGrad=false;}
    (junction 183) -> (junction 179)
    task_hold -> (junction 182) [order 1] : [EgoFol==0]
    (junction 182) -> (junction 158) [order 2]
    (junction 158) -> (junction 183) : {b_doGrad=false;
        | b_doQP=false;}
    (junction 179) -> (junction 175)
    (junction 182) -> (junction 156) [order 1] : [trigSQP==true]
    (junction 162) -> (junction 175)
    (junction 156) -> (junction 176)
    (junction 176) -> (junction 162) : {b_doGrad=true;
        | b_doQP=true;task_start_time = current_time;}
    (junction 175) -> (junction 190)
    (junction 160) -> (junction 190) : {task_start_time = current_time;}
    task_hold -> (junction 165) [order 2] : [trigSQP && EgoFol ]
    (junction 165) -> (junction 160) : {b_doGrad=true;
        | b_doQP=true;
        | b_exitQP=false;
        | b_termQP=false;}
    (junction 190) -> (junction 255)
    (junction 255) -> (junction 184)
    task_hold -> (junction 191) [order 3] : [EgoFol && E2C_stSolve && E2C_stGrad]
    (junction 191) -> (junction 188) [order 1] : [current_time-task_start_time<E2C_tiSolverPeriod_C-DeltaT]
    (junction 188) -> (junction 184) : {b_doGrad=false; b_doQP=true;
        | b_exitQP=false; }
    (junction 191) -> (junction 187) [order 2]
    (junction 184) -> (junction 185)
    (junction 187) -> (junction 185) : {b_exitQP=true; }
    (junction 185) -> (junction 171)
    task_hold -> (junction 186) [order 4] : [EgoFol && E2C_stSolve && E2C_stGrad==0]
    (junction 186) -> (junction 157) [order 1] : [current_time-task_start_time<E2C_tiSolverPeriod_C-DeltaT]
    (junction 157) -> (junction 171) : {b_doQP=true;b_exitQP=false;}
    (junction 186) -> (junction 189) [order 2]
    (junction 171) -> (junction 161)
    (junction 189) -> (junction 161) : {b_doQP=false; b_exitQP=true;}
    (junction 161) -> (junction 169)
    task_hold -> (junction 169) [order 5] : [EgoFol && E2C_stSolve ==0]
    (junction 169) -> (junction 167)
    task_hold -> (junction 167) [order 6]
    (junction 167) -> (junction 192)
    (junction 192) -> task_hold
  state solver_sched [parallel]
    settings: executionOrder=2
    state wait_next_task_1
      en: E2C_stSolve=false;
      E2C_stGrad=false;
    state Just_Got_grad
      en: E2C_stSolve=true;
      E2C_stGrad=true;
    state Solver_Running
      en: E2C_stSolve=true;
      E2C_stGrad=false;
    (default) -> (junction 145)
    (junction 145) -> (junction 148) [order 1] : [EgoFol==0 && b_doQP]
    wait_next_task_1 -> (junction 148) [order 2] : [EgoFol==0 && b_doQP]
    (junction 148) -> (junction 114) : {doGrad;doSolver;}
    (junction 145) -> wait_next_task_1 [order 2]
    wait_next_task_1 -> wait_next_task_1 [order 3]
    wait_next_task_1 -> (junction 140) [order 1] : [EgoFol && b_doGrad]
    (junction 140) -> (junction 132) : {doGrad;
        | solver_ctr= int8(0); }
    (junction 132) -> (junction 141) : {b_doGrad=false;
        | solver_start_time = current_time;
        | }
    (junction 141) -> (junction 115) : {
        | z_ref=zeros(41,1);
        | %z_ref(1:39)=z_laststep(2:40);
        | z_ref(1:39)=z_qp(2:40);
        | z_ref(41)=0;z_ref(40) = 0;
        | }
    (junction 115) -> (junction 133) : {doSolver; solver_ctr=solver_ctr+1;
        | %z_ref = z_qp;
        | }
    (junction 133) -> Just_Got_grad
    Just_Got_grad -> (junction 113)
    (junction 125) -> wait_next_task_1 : {solver_end_time = current_time;
        | send(SendDemand);}
    (junction 113) -> (junction 142) [order 2]
    (junction 142) -> Solver_Running : {z_ref = z_qp;}
    (junction 113) -> (junction 117) [order 1] : [b_doQP &&b_exitQP==0]
    (junction 114) -> (junction 150) : {z_ref = z_qp;}
    (junction 143) -> Solver_Running : {z_ref = z_qp;}
    (junction 134) -> (junction 143) : {
        | dz = max(abs(z_ref(1:40)-z_qp(1:40)));
        | b_termQP=(solver_ctr>=Max_iter) || ((dz<dz_term)&&(df<df_term));
        | % Add () for last two conditions
        | }
    (junction 117) -> (junction 134) : {doSolver; solver_ctr=solver_ctr+1;
        | %z_ref = z_qp;
        | }
    (junction 135) -> (junction 117)
    (junction 150) -> (junction 125)
    (junction 118) -> (junction 125)
    Solver_Running -> (junction 118) [order 2] : [b_doQP && b_exitQP]
    (junction 243) -> (junction 118)
    Solver_Running -> (junction 243) [order 3] : [b_doQP && b_termQP]
    (junction 246) -> (junction 243)
    Solver_Running -> (junction 246) [order 4]
    Solver_Running -> (junction 129) [order 1] : [b_doQP && b_exitQP==0 && b_termQP==0]
    (junction 129) -> (junction 135)
  data: trigSQP input boolean; current_time input single; E2C_tiSolverPeriod_C input single; EgoFol input boolean; Max_iter input int8; E2C_Delta_T input; dz_term input double; df_term input double; z_ref output; z_laststep input; z_qp input; delta_z local double; task_start_time local single; solver_ctr output int8; solver_start_time output single; solver_end_time output single; df input; b_doGrad local boolean; b_doQP local boolean; E2C_stGrad output boolean =false; DeltaT input; E2C_stSolve output boolean; b_exitQP output boolean; dz output; b_termQP output boolean
  events: doGrad output FUNCTION_CALL_EVENT; SendDemand output FUNCTION_CALL_EVENT; doSolver output FUNCTION_CALL_EVENT

== matlab function Solver/Function-Call Subsystem/MATLAB Function ==
  data: u input; y output
function y = fcn(u)

y = u;

== matlab function Solver/Send  V_demand/MATLAB send demand ==
  data: u input; y output
function y = fcn(u)

y = u;

== matlab function Solver/Send  V_demand/Triggered Subsystem/MATLAB Function1 ==
  data: V_OPT input; V_OUTPUT_step1_delayed input; pt_current input; V_Opt_array_modified output; V_OUTPUT_current_delayed input
function V_Opt_array_modified   = fcn(V_OPT,V_OUTPUT_step1_delayed,pt_current,V_OUTPUT_current_delayed)

V_Opt_array_modified = V_OPT;
%pt_current

V_Opt_array_modified(1)=V_OUTPUT_step1_delayed;
if pt_current >=1 && pt_current <= 40
V_Opt_array_modified(pt_current)=V_OUTPUT_current_delayed;
end
